simulink model "Timer"  (R2021b)
settings: Solver=ode3  StartTime=0.0  StopTime=10.0  FixedStep=0.01  RelTol=1e-3
settings Model: Creator=mwjae  LastModifiedBy=mwjae

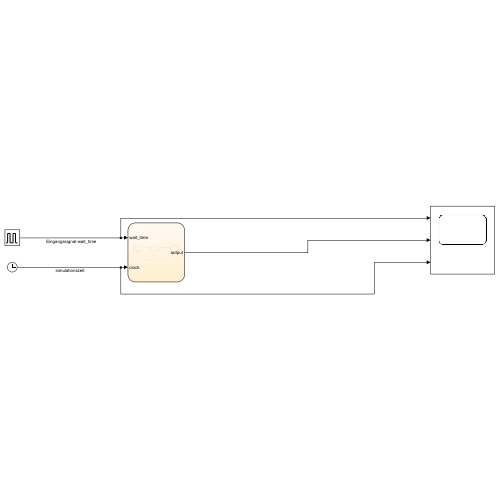
[thumbnail: Simulink's stored preview of the top-level diagram]
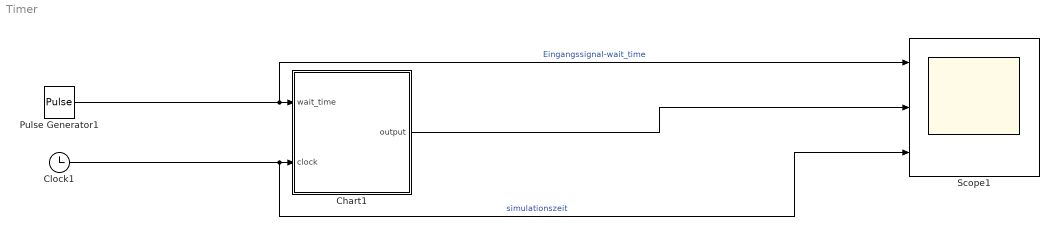
== system Timer ==
  Chart1 : Stateflow chart  TreatAsAtomicUnit=on
  Clock1 : Clock
  Pulse Generator1 : DiscretePulseGenerator  PulseType=Time based  Period=3  PulseWidth=50
  Scope1 : Scope  NumInputPorts=3
  wires:
  Chart1/1(output) -> Scope1/2
  Clock1/1 -> Chart1/2(clock), Scope1/3  "simulationszeit"
  Pulse Generator1/1 -> Scope1/1, Chart1/1(wait_time)  "Eingangssignal-wait_time"

== stateflow chart Timer/Chart1 ==
  state Output_zustand
    output =1 ;
  state wait_zustand
    output = 0;
  state wait_zustand1
  (default) -> wait_zustand
  wait_zustand1 -> Output_zustand : after(1,sec)
  wait_zustand -> wait_zustand1 : [wait_time == 1]
  Output_zustand -> wait_zustand : [output == 1]
  data: wait_time input; output output; clock input
